simulink model "agent_consensus"  (R2021b)
settings: Solver=VariableStepAuto  StartTime=0.0  StopTime=100  RelTol=1e-3
settings Model: Creator=Mahdi  LastModifiedBy=Mahdi

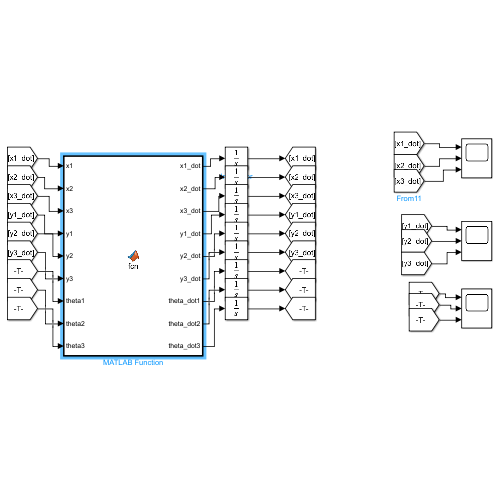
[thumbnail: Simulink's stored preview of the top-level diagram]
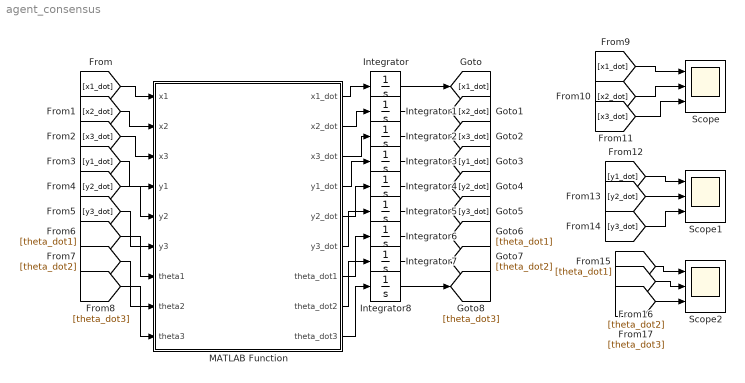
== system agent_consensus ==
  Integrator : Integrator  InitialCondition=rand(1,1)
  Integrator1 : Integrator  InitialCondition=rand(1,1)
  Integrator{2..8} (7 alike) : Integrator  InitialCondition=rand
  MATLAB Function : MATLAB Function  TreatAsAtomicUnit=on
  Scope : Scope  NumInputPorts=3
  Scope1 : Scope  NumInputPorts=3
  Scope2 : Scope  NumInputPorts=3
  wires:
  MATLAB Function/1(x1_dot) -> Integrator/1
  MATLAB Function/2(x2_dot) -> Integrator1/1
  MATLAB Function/3(x3_dot) -> Integrator2/1
  MATLAB Function/4(y1_dot) -> Integrator3/1
  MATLAB Function/5(y2_dot) -> Integrator4/1
  MATLAB Function/6(y3_dot) -> Integrator5/1
  MATLAB Function/7(theta_dot1) -> Integrator6/1
  MATLAB Function/8(theta_dot2) -> Integrator7/1
  MATLAB Function/9(theta_dot3) -> Integrator8/1
  Integrator/1 -> [x1_dot]
  Integrator1/1 -> [x2_dot]
  Integrator2/1 -> [x3_dot]
  Integrator3/1 -> [y1_dot]
  Integrator4/1 -> [y2_dot]
  Integrator5/1 -> [y3_dot]
  Integrator6/1 -> [theta_dot1]
  Integrator7/1 -> [theta_dot2]
  Integrator8/1 -> [theta_dot3]
  [x1_dot] -> MATLAB Function/1(x1)
  [x2_dot] -> MATLAB Function/2(x2)
  [x3_dot] -> MATLAB Function/3(x3)
  [y1_dot] -> MATLAB Function/4(y1)
  [y2_dot] -> MATLAB Function/5(y2)
  [y3_dot] -> MATLAB Function/6(y3)
  [theta_dot1] -> MATLAB Function/7(theta1)
  [theta_dot2] -> MATLAB Function/8(theta2)
  [theta_dot3] -> MATLAB Function/9(theta3)
  [x1_dot] -> Scope/1
  [x2_dot] -> Scope/2
  [x3_dot] -> Scope/3
  [y1_dot] -> Scope1/1
  [y2_dot] -> Scope1/2
  [y3_dot] -> Scope1/3
  [theta_dot3] -> Scope2/3
  [theta_dot2] -> Scope2/2
  [theta_dot1] -> Scope2/1

== matlab function agent_consensus/MATLAB Function ==
  data: x1 input; x1_dot output; x2 input; x3 input; y1 input; y2 input; y3 input; theta1 input; theta2 input; theta3 input; x2_dot output; x3_dot output; y1_dot output; y2_dot output; y3_dot output; theta_dot1 output; theta_dot2 output; theta_dot3 output
function [x1_dot, x2_dot, x3_dot, y1_dot, y2_dot, y3_dot, theta_dot1, theta_dot2, theta_dot3] = fcn(x1, x2, x3, y1 ,y2, y3, theta1, theta2,theta3)
xl1 = 1;
yl1 = 1;
thetal1 = 0;

% calculate Xdot

x1_dot = x2 - x1;
x2_dot = x3 - x2;
x3_dot = x1 - x3 + xl1 - x1;

%Calculate Ydot
y1_dot = y2 - y1;
y2_dot = y3 - y2;
y3_dot = y1 - y3 + yl1 - y1;

%Calculate thetadot
theta_dot1 = theta2 - theta1;
theta_dot2 = theta3 - theta2;
theta_dot3 = theta1 - theta3 + thetal1 - theta1;
